simulink model "TFlex_PID"  (R2018a)
settings: Solver=FixedStepDiscrete  StartTime=0.0  StopTime=t_end  FixedStep=ts  RelTol=1e-3
PreLoadFcn:
  | Ts = 0.001;
InitFcn:
  | Ts = 0.001;
values from neighbouring files (symbols this model uses):
  a0 = omega_n^3    (= 31006276.6803)    [Tflex_PID_init.m]
  a1 = 3*omega_n^2    (= 296088.132033)    [Tflex_PID_init.m]
  a2 = 3*omega_n    (= 942.477796077)    [Tflex_PID_init.m]
  b = ones(2*D,Q)*0.001    [Tflex_PID_init.m]
  D = 21    [Tflex_PID_init.m]
  I_limit_max = 500    [Tflex_PID_init.m]
  I_limit_min = -500    [Tflex_PID_init.m]
  Kd = kp*(tau_z-tau_p*(1+(tau_z+tau_p)/tau_i))    [Tflex_PID_init.m]
  Ki = kp/tau_i    [Tflex_PID_init.m]
  Kp = kp*(1+(tau_z-tau_p)/tau_i)    [Tflex_PID_init.m]
  kp = m_eq*crossOver^2/sqrt(1/alpha)    [Tflex_PID_init.m]
  R = eye(2*D,2*D)*sn^2    [Tflex_PID_init.m]
  sf = 185.90    (= 185.9)    [Tflex_PID_init.m]
  t_end = 200    [Tflex_PID_init.m]    (also in multisineInit.m = t(end))
  tau_i = beta*tau_z    [Tflex_PID_init.m]
  tau_p = 1/(crossOver*sqrt(1/alpha))    [Tflex_PID_init.m]
  tau_z = sqrt(1/alpha)/crossOver    [Tflex_PID_init.m]
  ts = 1/1000    (= 0.001)    [Tflex_PID_init.m]    (also in init.m = 0.00025; multisineInit.m)
  w = ones(2*D,Q)*0.001    [Tflex_PID_init.m]
undefined symbols (not defined in the file or in its folder): DiscIntNeverNeededParam, LPden, LPnum, SIGMA
libraries: xpcethercatlib x91, simulink x61, slrtlib x9
(part 2 of 2)

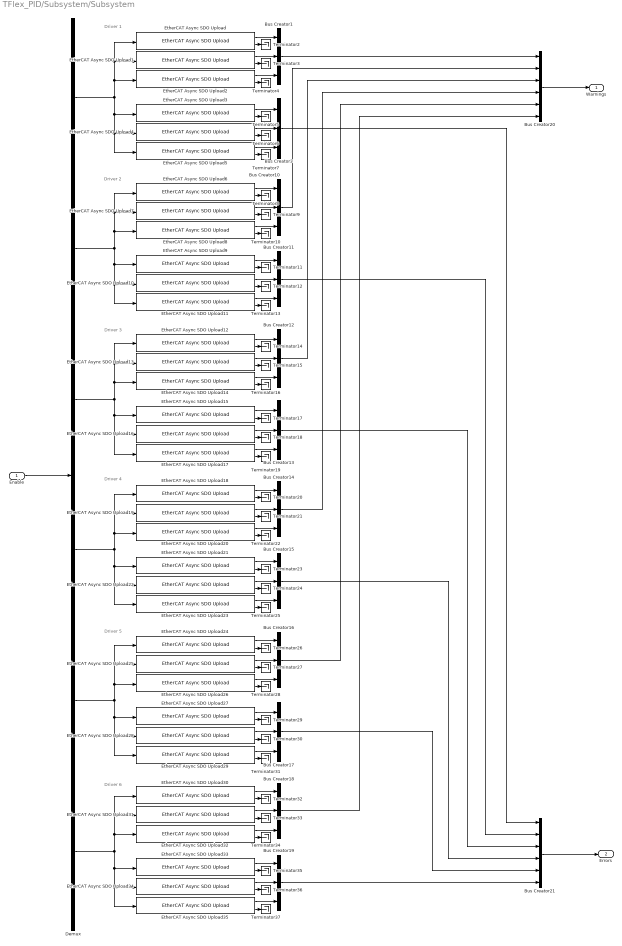
== system TFlex_PID/Subsystem/Subsystem ==
  note: Driver 1
  note: Driver 2
  note: Driver 3
  note: Driver 4
  note: Driver 5
  note: Driver 6
  Enable : Inport
  Bus Creator{1,3,10..19} (12 alike) : BusCreator  Inputs=3
  Bus Creator20 : BusCreator  Inputs=6
  Bus Creator21 : BusCreator  Inputs=6
  Demux : Demux  Outputs=6
  EtherCAT Async SDO Upload : xpcethercatlib/EtherCAT Async SDO Upload  index=8192  subIndex=1  sig_type=uint32  sig_dim=1  device_id=0  slave_name=Drive 2 (AKD)  sample_time=1  slave_addr=1001  selected_slave=Term 1 (EK1100)  timeout=500  slave_found=1
      settings: SourceProductName=Simulink Real-Time  SourceProductBaseCode=XP
  EtherCAT Async SDO Upload1 : xpcethercatlib/EtherCAT Async SDO Upload  index=8192  subIndex=2  sig_type=uint32  sig_dim=1  device_id=0  slave_name=Drive 2 (AKD)  sample_time=1  slave_addr=1001  selected_slave=Term 1 (EK1100)  timeout=500  slave_found=1
      settings: SourceProductName=Simulink Real-Time  SourceProductBaseCode=XP
  EtherCAT Async SDO Upload10 : xpcethercatlib/EtherCAT Async SDO Upload  index=8193  subIndex=2  sig_type=uint32  sig_dim=1  device_id=0  slave_name=Drive 3 (AKD)  sample_time=1  slave_addr=1002  selected_slave=Term 1 (EK1100)  timeout=500  slave_found=1
      settings: SourceProductName=Simulink Real-Time  SourceProductBaseCode=XP
  EtherCAT Async SDO Upload11 : xpcethercatlib/EtherCAT Async SDO Upload  index=8193  subIndex=3  sig_type=uint32  sig_dim=1  device_id=0  slave_name=Drive 3 (AKD)  sample_time=1  slave_addr=1002  selected_slave=Term 1 (EK1100)  timeout=500  slave_found=1
      settings: SourceProductName=Simulink Real-Time  SourceProductBaseCode=XP
  EtherCAT Async SDO Upload12 : xpcethercatlib/EtherCAT Async SDO Upload  index=8192  subIndex=1  sig_type=uint32  sig_dim=1  device_id=0  slave_name=Drive 4 (AKD)  sample_time=1  slave_addr=1003  selected_slave=Term 1 (EK1100)  timeout=500  slave_found=1
      settings: SourceProductName=Simulink Real-Time  SourceProductBaseCode=XP
  EtherCAT Async SDO Upload13 : xpcethercatlib/EtherCAT Async SDO Upload  index=8192  subIndex=2  sig_type=uint32  sig_dim=1  device_id=0  slave_name=Drive 4 (AKD)  sample_time=1  slave_addr=1003  selected_slave=Term 1 (EK1100)  timeout=500  slave_found=1
      settings: SourceProductName=Simulink Real-Time  SourceProductBaseCode=XP
  EtherCAT Async SDO Upload14 : xpcethercatlib/EtherCAT Async SDO Upload  index=8192  subIndex=3  sig_type=uint32  sig_dim=1  device_id=0  slave_name=Drive 4 (AKD)  sample_time=1  slave_addr=1003  selected_slave=Term 1 (EK1100)  timeout=500  slave_found=1
      settings: SourceProductName=Simulink Real-Time  SourceProductBaseCode=XP
  EtherCAT Async SDO Upload15 : xpcethercatlib/EtherCAT Async SDO Upload  index=8193  subIndex=1  sig_type=uint32  sig_dim=1  device_id=0  slave_name=Drive 4 (AKD)  sample_time=1  slave_addr=1003  selected_slave=Term 1 (EK1100)  timeout=500  slave_found=1
      settings: SourceProductName=Simulink Real-Time  SourceProductBaseCode=XP
  EtherCAT Async SDO Upload16 : xpcethercatlib/EtherCAT Async SDO Upload  index=8193  subIndex=2  sig_type=uint32  sig_dim=1  device_id=0  slave_name=Drive 4 (AKD)  sample_time=1  slave_addr=1003  selected_slave=Term 1 (EK1100)  timeout=500  slave_found=1
      settings: SourceProductName=Simulink Real-Time  SourceProductBaseCode=XP
  EtherCAT Async SDO Upload17 : xpcethercatlib/EtherCAT Async SDO Upload  index=8193  subIndex=3  sig_type=uint32  sig_dim=1  device_id=0  slave_name=Drive 4 (AKD)  sample_time=1  slave_addr=1003  selected_slave=Term 1 (EK1100)  timeout=500  slave_found=1
      settings: SourceProductName=Simulink Real-Time  SourceProductBaseCode=XP
  EtherCAT Async SDO Upload18 : xpcethercatlib/EtherCAT Async SDO Upload  index=8192  subIndex=1  sig_type=uint32  sig_dim=1  device_id=0  slave_name=Drive 5 (AKD)  sample_time=1  slave_addr=1004  selected_slave=Term 1 (EK1100)  timeout=500  slave_found=1
      settings: SourceProductName=Simulink Real-Time  SourceProductBaseCode=XP
  EtherCAT Async SDO Upload19 : xpcethercatlib/EtherCAT Async SDO Upload  index=8192  subIndex=2  sig_type=uint32  sig_dim=1  device_id=0  slave_name=Drive 5 (AKD)  sample_time=1  slave_addr=1004  selected_slave=Term 1 (EK1100)  timeout=500  slave_found=1
      settings: SourceProductName=Simulink Real-Time  SourceProductBaseCode=XP
  EtherCAT Async SDO Upload2 : xpcethercatlib/EtherCAT Async SDO Upload  index=8192  subIndex=3  sig_type=uint32  sig_dim=1  device_id=0  slave_name=Drive 1 (AKD)  sample_time=1  slave_addr=1001  selected_slave=Term 1 (EK1100)  timeout=500  slave_found=1
      settings: SourceProductName=Simulink Real-Time  SourceProductBaseCode=XP
  EtherCAT Async SDO Upload20 : xpcethercatlib/EtherCAT Async SDO Upload  index=8192  subIndex=3  sig_type=uint32  sig_dim=1  device_id=0  slave_name=Drive 5 (AKD)  sample_time=1  slave_addr=1004  selected_slave=Term 1 (EK1100)  timeout=500  slave_found=1
      settings: SourceProductName=Simulink Real-Time  SourceProductBaseCode=XP
  EtherCAT Async SDO Upload21 : xpcethercatlib/EtherCAT Async SDO Upload  index=8193  subIndex=1  sig_type=uint32  sig_dim=1  device_id=0  slave_name=Drive 5 (AKD)  sample_time=1  slave_addr=1004  selected_slave=Term 1 (EK1100)  timeout=500  slave_found=1
      settings: SourceProductName=Simulink Real-Time  SourceProductBaseCode=XP
  EtherCAT Async SDO Upload22 : xpcethercatlib/EtherCAT Async SDO Upload  index=8193  subIndex=2  sig_type=uint32  sig_dim=1  device_id=0  slave_name=Drive 5 (AKD)  sample_time=1  slave_addr=1004  selected_slave=Term 1 (EK1100)  timeout=500  slave_found=1
      settings: SourceProductName=Simulink Real-Time  SourceProductBaseCode=XP
  EtherCAT Async SDO Upload23 : xpcethercatlib/EtherCAT Async SDO Upload  index=8193  subIndex=3  sig_type=uint32  sig_dim=1  device_id=0  slave_name=Drive 5 (AKD)  sample_time=1  slave_addr=1004  selected_slave=Term 1 (EK1100)  timeout=500  slave_found=1
      settings: SourceProductName=Simulink Real-Time  SourceProductBaseCode=XP
  EtherCAT Async SDO Upload24 : xpcethercatlib/EtherCAT Async SDO Upload  index=8192  subIndex=1  sig_type=uint32  sig_dim=1  device_id=0  slave_name=Drive 6 (AKD)  sample_time=1  slave_addr=1005  selected_slave=Term 1 (EK1100)  timeout=500  slave_found=1
      settings: SourceProductName=Simulink Real-Time  SourceProductBaseCode=XP
  EtherCAT Async SDO Upload25 : xpcethercatlib/EtherCAT Async SDO Upload  index=8192  subIndex=2  sig_type=uint32  sig_dim=1  device_id=0  slave_name=Drive 6 (AKD)  sample_time=1  slave_addr=1005  selected_slave=Term 1 (EK1100)  timeout=500  slave_found=1
      settings: SourceProductName=Simulink Real-Time  SourceProductBaseCode=XP
  EtherCAT Async SDO Upload26 : xpcethercatlib/EtherCAT Async SDO Upload  index=8192  subIndex=3  sig_type=uint32  sig_dim=1  device_id=0  slave_name=Drive 6 (AKD)  sample_time=1  slave_addr=1005  selected_slave=Term 1 (EK1100)  timeout=500  slave_found=1
      settings: SourceProductName=Simulink Real-Time  SourceProductBaseCode=XP
  EtherCAT Async SDO Upload27 : xpcethercatlib/EtherCAT Async SDO Upload  index=8193  subIndex=1  sig_type=uint32  sig_dim=1  device_id=0  slave_name=Drive 6 (AKD)  sample_time=1  slave_addr=1005  selected_slave=Term 1 (EK1100)  timeout=500  slave_found=1
      settings: SourceProductName=Simulink Real-Time  SourceProductBaseCode=XP
  EtherCAT Async SDO Upload28 : xpcethercatlib/EtherCAT Async SDO Upload  index=8193  subIndex=2  sig_type=uint32  sig_dim=1  device_id=0  slave_name=Drive 6 (AKD)  sample_time=1  slave_addr=1005  selected_slave=Term 1 (EK1100)  timeout=500  slave_found=1
      settings: SourceProductName=Simulink Real-Time  SourceProductBaseCode=XP
  EtherCAT Async SDO Upload29 : xpcethercatlib/EtherCAT Async SDO Upload  index=8193  subIndex=3  sig_type=uint32  sig_dim=1  device_id=0  slave_name=Drive 6 (AKD)  sample_time=1  slave_addr=1005  selected_slave=Term 1 (EK1100)  timeout=500  slave_found=1
      settings: SourceProductName=Simulink Real-Time  SourceProductBaseCode=XP
  EtherCAT Async SDO Upload3 : xpcethercatlib/EtherCAT Async SDO Upload  index=8193  subIndex=1  sig_type=uint32  sig_dim=1  device_id=0  slave_name=""  sample_time=1  slave_addr=0  selected_slave=Term 1 (EK1100)  timeout=500  slave_found=1
      settings: SourceProductName=Simulink Real-Time  SourceProductBaseCode=XP
  EtherCAT Async SDO Upload30 : xpcethercatlib/EtherCAT Async SDO Upload  index=8192  subIndex=1  sig_type=uint32  sig_dim=1  device_id=0  slave_name=Drive 7 (AKD)  sample_time=1  slave_addr=1006  selected_slave=Term 1 (EK1100)  timeout=500  slave_found=1
      settings: SourceProductName=Simulink Real-Time  SourceProductBaseCode=XP
  EtherCAT Async SDO Upload31 : xpcethercatlib/EtherCAT Async SDO Upload  index=8192  subIndex=2  sig_type=uint32  sig_dim=1  device_id=0  slave_name=Drive 7 (AKD)  sample_time=1  slave_addr=1006  selected_slave=Term 1 (EK1100)  timeout=500  slave_found=1
      settings: SourceProductName=Simulink Real-Time  SourceProductBaseCode=XP
  EtherCAT Async SDO Upload32 : xpcethercatlib/EtherCAT Async SDO Upload  index=8192  subIndex=3  sig_type=uint32  sig_dim=1  device_id=0  slave_name=Drive 7 (AKD)  sample_time=1  slave_addr=1006  selected_slave=Term 1 (EK1100)  timeout=500  slave_found=1
      settings: SourceProductName=Simulink Real-Time  SourceProductBaseCode=XP
  EtherCAT Async SDO Upload33 : xpcethercatlib/EtherCAT Async SDO Upload  index=8193  subIndex=1  sig_type=uint32  sig_dim=1  device_id=0  slave_name=Drive 7 (AKD)  sample_time=1  slave_addr=1006  selected_slave=Term 1 (EK1100)  timeout=500  slave_found=1
      settings: SourceProductName=Simulink Real-Time  SourceProductBaseCode=XP
  EtherCAT Async SDO Upload34 : xpcethercatlib/EtherCAT Async SDO Upload  index=8193  subIndex=2  sig_type=uint32  sig_dim=1  device_id=0  slave_name=Drive 7 (AKD)  sample_time=1  slave_addr=1006  selected_slave=Term 1 (EK1100)  timeout=500  slave_found=1
      settings: SourceProductName=Simulink Real-Time  SourceProductBaseCode=XP
  EtherCAT Async SDO Upload35 : xpcethercatlib/EtherCAT Async SDO Upload  index=8193  subIndex=3  sig_type=uint32  sig_dim=1  device_id=0  slave_name=Drive 7 (AKD)  sample_time=1  slave_addr=1006  selected_slave=Term 1 (EK1100)  timeout=500  slave_found=1
      settings: SourceProductName=Simulink Real-Time  SourceProductBaseCode=XP
  EtherCAT Async SDO Upload4 : xpcethercatlib/EtherCAT Async SDO Upload  index=8193  subIndex=2  sig_type=uint32  sig_dim=1  device_id=0  slave_name=Drive 2 (AKD)  sample_time=1  slave_addr=1001  selected_slave=Term 1 (EK1100)  timeout=500  slave_found=1
      settings: SourceProductName=Simulink Real-Time  SourceProductBaseCode=XP
  EtherCAT Async SDO Upload5 : xpcethercatlib/EtherCAT Async SDO Upload  index=8193  subIndex=3  sig_type=uint32  sig_dim=1  device_id=0  slave_name=Drive 1 (AKD)  sample_time=1  slave_addr=1001  selected_slave=Term 1 (EK1100)  timeout=500  slave_found=1
      settings: SourceProductName=Simulink Real-Time  SourceProductBaseCode=XP
  EtherCAT Async SDO Upload6 : xpcethercatlib/EtherCAT Async SDO Upload  index=8192  subIndex=1  sig_type=uint32  sig_dim=1  device_id=0  slave_name=Drive 3 (AKD)  sample_time=1  slave_addr=1002  selected_slave=Term 1 (EK1100)  timeout=500  slave_found=1
      settings: SourceProductName=Simulink Real-Time  SourceProductBaseCode=XP
  EtherCAT Async SDO Upload7 : xpcethercatlib/EtherCAT Async SDO Upload  index=8192  subIndex=2  sig_type=uint32  sig_dim=1  device_id=0  slave_name=Drive 3 (AKD)  sample_time=1  slave_addr=1002  selected_slave=Term 1 (EK1100)  timeout=500  slave_found=1
      settings: SourceProductName=Simulink Real-Time  SourceProductBaseCode=XP
  EtherCAT Async SDO Upload8 : xpcethercatlib/EtherCAT Async SDO Upload  index=8192  subIndex=3  sig_type=uint32  sig_dim=1  device_id=0  slave_name=Drive 3 (AKD)  sample_time=1  slave_addr=1002  selected_slave=Term 1 (EK1100)  timeout=500  slave_found=1
      settings: SourceProductName=Simulink Real-Time  SourceProductBaseCode=XP
  EtherCAT Async SDO Upload9 : xpcethercatlib/EtherCAT Async SDO Upload  index=8193  subIndex=1  sig_type=uint32  sig_dim=1  device_id=0  slave_name=Drive 3 (AKD)  sample_time=1  slave_addr=1002  selected_slave=Term 1 (EK1100)  timeout=500  slave_found=1
      settings: SourceProductName=Simulink Real-Time  SourceProductBaseCode=XP
  Terminator{2..37} (36 alike) : Terminator
  Warnings : Outport
  Errors : Outport  Port=2
  wires:
  EtherCAT Async SDO Upload13/2 -> Terminator15/1
  EtherCAT Async SDO Upload23/2 -> Terminator25/1
  EtherCAT Async SDO Upload25/2 -> Terminator27/1
  EtherCAT Async SDO Upload9/2 -> Terminator11/1
  EtherCAT Async SDO Upload5/2 -> Terminator7/1
  EtherCAT Async SDO Upload30/2 -> Terminator32/1
  EtherCAT Async SDO Upload27/2 -> Terminator29/1
  EtherCAT Async SDO Upload12/2 -> Terminator14/1
  EtherCAT Async SDO Upload24/2 -> Terminator26/1
  EtherCAT Async SDO Upload26/2 -> Terminator28/1
  Bus Creator12/1 -> Bus Creator20/3
  Demux/3 -> EtherCAT Async SDO Upload12/1, EtherCAT Async SDO Upload13/1, EtherCAT Async SDO Upload14/1, EtherCAT Async SDO Upload17/1, EtherCAT Async SDO Upload16/1, EtherCAT Async SDO Upload15/1
  EtherCAT Async SDO Upload30/1 -> Bus Creator18/1
  Demux/2 -> EtherCAT Async SDO Upload11/1, EtherCAT Async SDO Upload10/1, EtherCAT Async SDO Upload9/1, EtherCAT Async SDO Upload6/1, EtherCAT Async SDO Upload7/1, EtherCAT Async SDO Upload8/1
  EtherCAT Async SDO Upload9/1 -> Bus Creator11/1
  EtherCAT Async SDO Upload18/2 -> Terminator20/1
  EtherCAT Async SDO Upload8/2 -> Terminator10/1
  EtherCAT Async SDO Upload11/2 -> Terminator13/1
  Demux/6 -> EtherCAT Async SDO Upload30/1, EtherCAT Async SDO Upload31/1, EtherCAT Async SDO Upload32/1, EtherCAT Async SDO Upload35/1, EtherCAT Async SDO Upload34/1, EtherCAT Async SDO Upload33/1
  Demux/4 -> EtherCAT Async SDO Upload18/1, EtherCAT Async SDO Upload19/1, EtherCAT Async SDO Upload20/1, EtherCAT Async SDO Upload23/1, EtherCAT Async SDO Upload22/1, EtherCAT Async SDO Upload21/1
  EtherCAT Async SDO Upload19/2 -> Terminator21/1
  Bus Creator19/1 -> Bus Creator21/6
  Demux/1 -> EtherCAT Async SDO Upload5/1, EtherCAT Async SDO Upload4/1, EtherCAT Async SDO Upload3/1, EtherCAT Async SDO Upload/1, EtherCAT Async SDO Upload1/1, EtherCAT Async SDO Upload2/1
  EtherCAT Async SDO Upload15/2 -> Terminator17/1
  Bus Creator14/1 -> Bus Creator20/4
  EtherCAT Async SDO Upload34/2 -> Terminator36/1
  Demux/5 -> EtherCAT Async SDO Upload24/1, EtherCAT Async SDO Upload25/1, EtherCAT Async SDO Upload26/1, EtherCAT Async SDO Upload29/1, EtherCAT Async SDO Upload28/1, EtherCAT Async SDO Upload27/1
  EtherCAT Async SDO Upload6/2 -> Terminator8/1
  EtherCAT Async SDO Upload/1 -> Bus Creator1/1
  EtherCAT Async SDO Upload7/2 -> Terminator9/1
  EtherCAT Async SDO Upload16/2 -> Terminator18/1
  Bus Creator13/1 -> Bus Creator21/3
  EtherCAT Async SDO Upload10/2 -> Terminator12/1
  EtherCAT Async SDO Upload35/2 -> Terminator37/1
  EtherCAT Async SDO Upload21/1 -> Bus Creator15/1
  Bus Creator16/1 -> Bus Creator20/5
  EtherCAT Async SDO Upload31/2 -> Terminator33/1
  EtherCAT Async SDO Upload32/1 -> Bus Creator18/3
  EtherCAT Async SDO Upload15/1 -> Bus Creator13/1
  EtherCAT Async SDO Upload/2 -> Terminator2/1
  EtherCAT Async SDO Upload13/1 -> Bus Creator12/2
  EtherCAT Async SDO Upload33/2 -> Terminator35/1
  EtherCAT Async SDO Upload4/2 -> Terminator6/1
  EtherCAT Async SDO Upload28/2 -> Terminator30/1
  EtherCAT Async SDO Upload1/2 -> Terminator3/1
  Bus Creator10/1 -> Bus Creator20/2
  EtherCAT Async SDO Upload8/1 -> Bus Creator10/3
  EtherCAT Async SDO Upload19/1 -> Bus Creator14/2
  EtherCAT Async SDO Upload20/2 -> Terminator22/1
  EtherCAT Async SDO Upload12/1 -> Bus Creator12/1
  EtherCAT Async SDO Upload29/2 -> Terminator31/1
  EtherCAT Async SDO Upload2/1 -> Bus Creator1/3
  EtherCAT Async SDO Upload26/1 -> Bus Creator16/3
  EtherCAT Async SDO Upload22/2 -> Terminator24/1
  EtherCAT Async SDO Upload28/1 -> Bus Creator17/2
  Bus Creator1/1 -> Bus Creator20/1
  EtherCAT Async SDO Upload3/2 -> Terminator5/1
  Bus Creator17/1 -> Bus Creator21/5
  EtherCAT Async SDO Upload2/2 -> Terminator4/1
  EtherCAT Async SDO Upload33/1 -> Bus Creator19/1
  EtherCAT Async SDO Upload17/1 -> Bus Creator13/3
  EtherCAT Async SDO Upload31/1 -> Bus Creator18/2
  EtherCAT Async SDO Upload27/1 -> Bus Creator17/1
  EtherCAT Async SDO Upload1/1 -> Bus Creator1/2
  EtherCAT Async SDO Upload3/1 -> Bus Creator3/1
  EtherCAT Async SDO Upload11/1 -> Bus Creator11/3
  EtherCAT Async SDO Upload7/1 -> Bus Creator10/2
  EtherCAT Async SDO Upload6/1 -> Bus Creator10/1
  EtherCAT Async SDO Upload34/1 -> Bus Creator19/2
  Bus Creator18/1 -> Bus Creator20/6
  EtherCAT Async SDO Upload22/1 -> Bus Creator15/2
  EtherCAT Async SDO Upload23/1 -> Bus Creator15/3
  EtherCAT Async SDO Upload18/1 -> Bus Creator14/1
  EtherCAT Async SDO Upload10/1 -> Bus Creator11/2
  EtherCAT Async SDO Upload14/1 -> Bus Creator12/3
  EtherCAT Async SDO Upload35/1 -> Bus Creator19/3
  EtherCAT Async SDO Upload24/1 -> Bus Creator16/1
  EtherCAT Async SDO Upload20/1 -> Bus Creator14/3
  Bus Creator3/1 -> Bus Creator21/1
  EtherCAT Async SDO Upload4/1 -> Bus Creator3/2
  EtherCAT Async SDO Upload25/1 -> Bus Creator16/2
  EtherCAT Async SDO Upload16/1 -> Bus Creator13/2
  Bus Creator15/1 -> Bus Creator21/4
  Bus Creator11/1 -> Bus Creator21/2
  EtherCAT Async SDO Upload5/1 -> Bus Creator3/3
  EtherCAT Async SDO Upload32/2 -> Terminator34/1
  EtherCAT Async SDO Upload29/1 -> Bus Creator17/3
  EtherCAT Async SDO Upload14/2 -> Terminator16/1
  EtherCAT Async SDO Upload17/2 -> Terminator19/1
  EtherCAT Async SDO Upload21/2 -> Terminator23/1
  Bus Creator21/1 -> Errors/1
  Bus Creator20/1 -> Warnings/1
  Enable/1 -> Demux/1

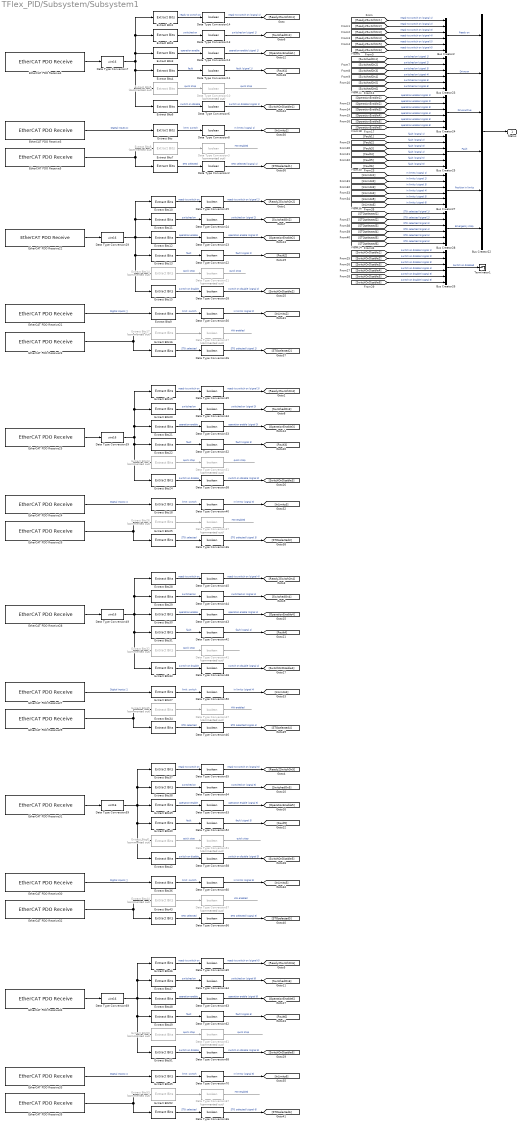
== system TFlex_PID/Subsystem/Subsystem1 ==
  Bus Creator2 : BusCreator  Inputs=ready to switch on (signal 1),ready to switch on (signal 2),ready to switch on (signal 3),ready to switch on (signal 4),ready to switch on (signal 5),ready to switch on (signal 6)
  Bus Creator22 : BusCreator  Inputs=Ready on,Drive on,Drive active,Fault,Position in limits,Emergency stop
  Bus Creator23 : BusCreator  Inputs=switched on (signal 1),switched on (signal 2),switched on (signal 3),switched on (signal 4),switched on (signal 5),switched on (signal 6)
  Bus Creator24 : BusCreator  Inputs=operation enable (signal 1),operation enable (signal 2),operation enable (signal 3),operation enable (signal 4),operation enable (signal 5),operation enable (signal 6)
  Bus Creator25 : BusCreator  Inputs=fault (signal 1),fault (signal 2),fault (signal 3),fault (signal 4),fault (signal 5),fault (signal 6)
  Bus Creator26 : BusCreator  Inputs=switch on disable (signal 1),switch on disable (signal 2),switch on disable (signal 3),switch on disable (signal 4),switch on disable (signal 5),switch on disable (signal 6)
  Bus Creator27 : BusCreator  Inputs=in limits (signal 1),in limits (signal 2),in limits (signal 3),in limits (signal 4),in limits (signal 5),in limits (signal 6)
  Bus Creator28 : BusCreator  Inputs=STO selected (signal 1),STO selected (signal 2),STO selected (signal 3),STO selected (signal 4),STO selected (signal 5),STO selected (signal 6)
  Data Type Conversion{3,10,21,27,31,37,41,47,51,57,61,67} (12 alike) : DataTypeConversion  Commented=on  OutDataTypeStr=boolean
  Data Type Conversion{2,6,8,11..14,22..26,28,30,32..36,38,40,42..46,48,50,52..56,58,60,62..66,68,70} (42 alike) : DataTypeConversion  OutDataTypeStr=boolean
  Data Type Conversion{7,29,39,49,59,69} (6 alike) : DataTypeConversion  OutDataTypeStr=uint16  RndMeth=Round
  EtherCAT PDO Receive21 : xpcethercatlib/EtherCAT PDO Receive  Priority=2  sig_name=Drive 3 (AKD).Inputs.Digital inputs  sig_offset=12528  sig_type=uint32  type_size=32  sig_dim=1  device_id=0  sample_time=0.001000
      settings: SourceProductName=Simulink Real-Time  SourceProductBaseCode=XP
  EtherCAT PDO Receive22 : xpcethercatlib/EtherCAT PDO Receive  Priority=2  sig_name=Drive 3 (AKD).Inputs.Statusword  sig_offset=12496  sig_type=uint16  type_size=16  sig_dim=1  device_id=0  sample_time=0.001000
      settings: SourceProductName=Simulink Real-Time  SourceProductBaseCode=XP
  EtherCAT PDO Receive23 : xpcethercatlib/EtherCAT PDO Receive  Priority=2  sig_name=Drive 3 (AKD).Inputs_2.Manufacturer status register  sig_offset=12624  sig_type=uint32  type_size=32  sig_dim=1  device_id=0  sample_time=0.001000
      settings: SourceProductName=Simulink Real-Time  SourceProductBaseCode=XP
  EtherCAT PDO Receive24 : xpcethercatlib/EtherCAT PDO Receive  Priority=2  sig_name=Drive 4 (AKD).Inputs.Digital inputs  sig_offset=24816  sig_type=uint32  type_size=32  sig_dim=1  device_id=0  sample_time=0.001000
      settings: SourceProductName=Simulink Real-Time  SourceProductBaseCode=XP
  EtherCAT PDO Receive25 : xpcethercatlib/EtherCAT PDO Receive  Priority=2  sig_name=Drive 4 (AKD).Inputs.Statusword  sig_offset=24784  sig_type=uint16  type_size=16  sig_dim=1  device_id=0  sample_time=0.001000
      settings: SourceProductName=Simulink Real-Time  SourceProductBaseCode=XP
  EtherCAT PDO Receive26 : xpcethercatlib/EtherCAT PDO Receive  Priority=2  sig_name=Drive 4 (AKD).Inputs_2.Manufacturer status register  sig_offset=24912  sig_type=uint32  type_size=32  sig_dim=1  device_id=0  sample_time=0.001000
      settings: SourceProductName=Simulink Real-Time  SourceProductBaseCode=XP
  EtherCAT PDO Receive27 : xpcethercatlib/EtherCAT PDO Receive  Priority=2  sig_name=Drive 5 (AKD).Inputs.Digital inputs  sig_offset=37104  sig_type=uint32  type_size=32  sig_dim=1  device_id=0  sample_time=0.001000
      settings: SourceProductName=Simulink Real-Time  SourceProductBaseCode=XP
  EtherCAT PDO Receive28 : xpcethercatlib/EtherCAT PDO Receive  Priority=2  sig_name=Drive 5 (AKD).Inputs.Statusword  sig_offset=37072  sig_type=uint16  type_size=16  sig_dim=1  device_id=0  sample_time=0.001000
      settings: SourceProductName=Simulink Real-Time  SourceProductBaseCode=XP
  EtherCAT PDO Receive29 : xpcethercatlib/EtherCAT PDO Receive  Priority=2  sig_name=Drive 5 (AKD).Inputs_2.Manufacturer status register  sig_offset=37200  sig_type=uint32  type_size=32  sig_dim=1  device_id=0  sample_time=0.001000
      settings: SourceProductName=Simulink Real-Time  SourceProductBaseCode=XP
  EtherCAT PDO Receive3 : xpcethercatlib/EtherCAT PDO Receive  Priority=2  sig_name=Drive 2 (AKD).Inputs.Digital inputs  sig_offset=496  sig_type=uint32  type_size=32  sig_dim=1  device_id=0  sample_time=0.001000
      settings: SourceProductName=Simulink Real-Time  SourceProductBaseCode=XP
  EtherCAT PDO Receive30 : xpcethercatlib/EtherCAT PDO Receive  Priority=2  sig_name=Drive 6 (AKD).Inputs.Digital inputs  sig_offset=37264  sig_type=uint32  type_size=32  sig_dim=1  device_id=0  sample_time=0.001000
      settings: SourceProductName=Simulink Real-Time  SourceProductBaseCode=XP
  EtherCAT PDO Receive31 : xpcethercatlib/EtherCAT PDO Receive  Priority=2  sig_name=Drive 6 (AKD).Inputs.Statusword  sig_offset=37232  sig_type=uint16  type_size=16  sig_dim=1  device_id=0  sample_time=0.001000
      settings: SourceProductName=Simulink Real-Time  SourceProductBaseCode=XP
  EtherCAT PDO Receive32 : xpcethercatlib/EtherCAT PDO Receive  Priority=2  sig_name=Drive 6 (AKD).Inputs_2.Manufacturer status register  sig_offset=37360  sig_type=uint32  type_size=32  sig_dim=1  device_id=0  sample_time=0.001000
      settings: SourceProductName=Simulink Real-Time  SourceProductBaseCode=XP
  EtherCAT PDO Receive33 : xpcethercatlib/EtherCAT PDO Receive  Priority=2  sig_name=Drive 7 (AKD).Inputs.Digital inputs  sig_offset=37424  sig_type=uint32  type_size=32  sig_dim=1  device_id=0  sample_time=0.001000
      settings: SourceProductName=Simulink Real-Time  SourceProductBaseCode=XP
  EtherCAT PDO Receive34 : xpcethercatlib/EtherCAT PDO Receive  Priority=2  sig_name=Drive 7 (AKD).Inputs.Statusword  sig_offset=37392  sig_type=uint16  type_size=16  sig_dim=1  device_id=0  sample_time=0.001000
      settings: SourceProductName=Simulink Real-Time  SourceProductBaseCode=XP
  EtherCAT PDO Receive35 : xpcethercatlib/EtherCAT PDO Receive  Priority=2  sig_name=Drive 7 (AKD).Inputs_2.Manufacturer status register  sig_offset=37520  sig_type=uint32  type_size=32  sig_dim=1  device_id=0  sample_time=0.001000
      settings: SourceProductName=Simulink Real-Time  SourceProductBaseCode=XP
  EtherCAT PDO Receive4 : xpcethercatlib/EtherCAT PDO Receive  Priority=2  sig_name=Drive 2 (AKD).Inputs.Statusword  sig_offset=464  sig_type=uint16  type_size=16  sig_dim=1  device_id=0  sample_time=0.001000
      settings: SourceProductName=Simulink Real-Time  SourceProductBaseCode=XP
  EtherCAT PDO Receive5 : xpcethercatlib/EtherCAT PDO Receive  Priority=2  sig_name=Drive 2 (AKD).Inputs_2.Manufacturer status register  sig_offset=592  sig_type=uint32  type_size=32  sig_dim=1  device_id=0  sample_time=0.001000
      settings: SourceProductName=Simulink Real-Time  SourceProductBaseCode=XP
  Extract Bits{,9,18,27,36,45} (6 alike) : simulink/Logic and Bit Operations/Extract Bits  bitsToExtract=Range of bits  numBits=8  bitIdxRange=[16]  outScalingMode=Treat bit field as an integer
      settings: SourceProductName=Simulink
  Extract Bits{1,10,19,28,37,46} (6 alike) : simulink/Logic and Bit Operations/Extract Bits  bitsToExtract=Range of bits  numBits=8  bitIdxRange=[0]  outScalingMode=Treat bit field as an integer
      settings: SourceProductName=Simulink
  Extract Bits{2,11,20,29,38,47} (6 alike) : simulink/Logic and Bit Operations/Extract Bits  bitsToExtract=Range of bits  numBits=8  bitIdxRange=[1]  outScalingMode=Treat bit field as an integer
      settings: SourceProductName=Simulink
  Extract Bits{3,12,21,30,39,48} (6 alike) : simulink/Logic and Bit Operations/Extract Bits  bitsToExtract=Range of bits  numBits=8  bitIdxRange=[2]  outScalingMode=Treat bit field as an integer
      settings: SourceProductName=Simulink
  Extract Bits{4,13,22,31,40,49} (6 alike) : simulink/Logic and Bit Operations/Extract Bits  bitsToExtract=Range of bits  numBits=8  bitIdxRange=[3]  outScalingMode=Treat bit field as an integer
      settings: SourceProductName=Simulink
  Extract Bits{5,14,23,32,41,50} (6 alike) : simulink/Logic and Bit Operations/Extract Bits  Commented=on  bitsToExtract=Range of bits  numBits=8  bitIdxRange=[5]  outScalingMode=Treat bit field as an integer
      settings: SourceProductName=Simulink
  Extract Bits{6,15,24,33,42,51} (6 alike) : simulink/Logic and Bit Operations/Extract Bits  bitsToExtract=Range of bits  numBits=8  bitIdxRange=[6]  outScalingMode=Treat bit field as an integer
      settings: SourceProductName=Simulink
  Extract Bits{7,16,25,34,43,52} (6 alike) : simulink/Logic and Bit Operations/Extract Bits  bitsToExtract=Range of bits  numBits=8  bitIdxRange=[13]  outScalingMode=Treat bit field as an integer
      settings: SourceProductName=Simulink
  Extract Bits{8,17,26,35,44,53} (6 alike) : simulink/Logic and Bit Operations/Extract Bits  Commented=on  bitsToExtract=Range of bits  numBits=8  bitIdxRange=[29]  outScalingMode=Treat bit field as an integer
      settings: SourceProductName=Simulink
  Terminator1 : Terminator
  Status : Outport
  wires:
  EtherCAT PDO Receive27/1 -> Extract Bits27/1  "Digital inputs []"
  [OperationEnable1] -> Bus Creator24/1  "operation enable (signal 1)"
  Data Type Conversion49/1 -> Extract Bits30/1, Extract Bits31/1, Extract Bits33/1, Extract Bits32/1, Extract Bits28/1, Extract Bits29/1
  [SwitchOnDisable3] -> Bus Creator26/3  "switch on disable (signal 3)"
  Data Type Conversion60/1 -> [InLimits5]  "in limits (signal 5)"
  EtherCAT PDO Receive26/1 -> Extract Bits26/1, Extract Bits25/1
  [OperationEnable2] -> Bus Creator24/2  "operation enable (signal 2)"
  [Fault2] -> Bus Creator25/2  "fault (signal 2)"
  Data Type Conversion31/1 -> ?  "quick stop"
  Data Type Conversion39/1 -> Extract Bits22/1, Extract Bits23/1, Extract Bits24/1, Extract Bits21/1, Extract Bits19/1, Extract Bits20/1
  Data Type Conversion69/1 -> Extract Bits51/1, Extract Bits50/1, Extract Bits49/1, Extract Bits46/1, Extract Bits47/1, Extract Bits48/1
  EtherCAT PDO Receive31/1 -> Data Type Conversion59/1
  Data Type Conversion68/1 -> [SwitchOnDisable6]  "switch on disable (signal 6)"
  [Ready2SwitchOn2] -> Bus Creator2/2  "ready to switch on (signal 2)"
  Extract Bits8/1 -> Data Type Conversion3/1
  Data Type Conversion7/1 -> Extract Bits1/1, Extract Bits2/1, Extract Bits3/1, Extract Bits6/1, Extract Bits5/1, Extract Bits4/1
  [SwitchOnDisable1] -> Bus Creator26/1  "switch on disable (signal 1)"
  Data Type Conversion50/1 -> [InLimits4]  "in limits (signal 4)"
  Data Type Conversion29/1 -> Extract Bits15/1, Extract Bits14/1, Extract Bits13/1, Extract Bits10/1, Extract Bits11/1, Extract Bits12/1
  Data Type Conversion51/1 -> ?  "quick stop"
  [STOselected4] -> Bus Creator28/4  "STO selected (signal 4)"
  Data Type Conversion13/1 -> [SwitchedOn1]  "switched on (signal 1)"
  Data Type Conversion43/1 -> [OperationEnable4]  "operation enable (signal 4)"
  Extract Bits44/1 -> Data Type Conversion57/1
  Bus Creator2/1 -> Bus Creator22/1  "Ready on"
  Extract Bits5/1 -> Data Type Conversion10/1  "quick stop"
  Data Type Conversion59/1 -> Extract Bits42/1, Extract Bits41/1, Extract Bits40/1, Extract Bits37/1, Extract Bits38/1, Extract Bits39/1
  Extract Bits24/1 -> Data Type Conversion38/1  "switch on disable"
  Data Type Conversion26/1 -> [STOselected2]  "STO selected (signal 2)"
  EtherCAT PDO Receive29/1 -> Extract Bits34/1, Extract Bits35/1
  Data Type Conversion63/1 -> [OperationEnable6]  "operation enable (signal 6)"
  Extract Bits36/1 -> Data Type Conversion60/1  "limit  switch"
  [Ready2SwitchOn5] -> Bus Creator2/5  "ready to switch on (signal 5)"
  Extract Bits35/1 -> Data Type Conversion47/1
  Data Type Conversion11/1 -> [Fault1]  "fault (signal 1)"
  Data Type Conversion58/1 -> [SwitchOnDisable5]  "switch on disable (signal 5)"
  Extract Bits48/1 -> Data Type Conversion63/1  "operation enable"
  Data Type Conversion35/1 -> [Ready2SwitchOn3]  "ready to switch on (signal 3)"
  EtherCAT PDO Receive23/1 -> Extract Bits17/1, Extract Bits16/1
  Data Type Conversion55/1 -> [Ready2SwitchOn5]  "ready to switch on (signal 5)"
  [Fault6] -> Bus Creator25/6  "fault (signal 6)"
  [SwitchedOn3] -> Bus Creator23/3  "switched on (signal 3)"
  Data Type Conversion54/1 -> [SwitchedOn5]  "switched on (signal 5)"
  [InLimits3] -> Bus Creator27/3  "in limits (signal 3)"
  Data Type Conversion2/1 -> [STOselected1]  "STO selected (signal 1)"
  [STOselected6] -> Bus Creator28/6  "STO selected (signal 6)"
  Extract Bits46/1 -> Data Type Conversion65/1  "ready to switch on"
  [SwitchOnDisable2] -> Bus Creator26/2  "switch on disable (signal 2)"
  Data Type Conversion64/1 -> [SwitchedOn6]  "switched on (signal 6)"
  [InLimits4] -> Bus Creator27/4  "in limits (signal 4)"
  Data Type Conversion70/1 -> [InLimits6]  "in limits (signal 6)"
  [SwitchedOn5] -> Bus Creator23/5  "switched on (signal 5)"
  [STOselected5] -> Bus Creator28/5  "STO selected (signal 5)"
  [InLimits6] -> Bus Creator27/6  "in limits (signal 6)"
  EtherCAT PDO Receive32/1 -> Extract Bits43/1, Extract Bits44/1
  Data Type Conversion65/1 -> [Ready2SwitchOn6]  "ready to switch on (signal 6)"
  [OperationEnable3] -> Bus Creator24/3  "operation enable (signal 3)"
  Data Type Conversion48/1 -> [SwitchOnDisable4]  "switch on disable (signal 4)"
  Data Type Conversion32/1 -> [Fault3]  "fault (signal 3)"
  Data Type Conversion46/1 -> [STOselected4]  "STO selected (signal 4)"
  Data Type Conversion38/1 -> [SwitchOnDisable3]  "switch on disable (signal 3)"
  Data Type Conversion23/1 -> [OperationEnable2]  "operation enable (signal 2)"
  Extract Bits39/1 -> Data Type Conversion53/1  "operation enable"
  [SwitchedOn4] -> Bus Creator23/4  "switched on (signal 4)"
  Extract Bits38/1 -> Data Type Conversion54/1  "switched on"
  [STOselected2] -> Bus Creator28/2  "STO selected (signal 2)"
  Data Type Conversion34/1 -> [SwitchedOn3]  "switched on (signal 3)"
  Extract Bits3/1 -> Data Type Conversion12/1  "operation enable"
  Data Type Conversion45/1 -> [Ready2SwitchOn4]  "ready to switch on (signal 4)"
  Extract Bits43/1 -> Data Type Conversion56/1  "STO selected"
  Data Type Conversion8/1 -> [InLimits1]  "in limits (signal 1)"
  [Ready2SwitchOn4] -> Bus Creator2/4  "ready to switch on (signal 4)"
  [STOselected3] -> Bus Creator28/3  "STO selected (signal 3)"
  [STOselected1] -> Bus Creator28/1  "STO selected (signal 1)"
  [InLimits5] -> Bus Creator27/5  "in limits (signal 5)"
  Bus Creator27/1 -> Bus Creator22/5  "Position in limits"
  Data Type Conversion33/1 -> [OperationEnable3]  "operation enable (signal 3)"
  Extract Bits14/1 -> Data Type Conversion21/1  "quick stop"
  Extract Bits45/1 -> Data Type Conversion70/1  "limit  switch"
  [Fault1] -> Bus Creator25/1  "fault (signal 1)"
  EtherCAT PDO Receive4/1 -> Data Type Conversion7/1
  Data Type Conversion40/1 -> [InLimits3]  "in limits (signal 3)"
  Extract Bits47/1 -> Data Type Conversion64/1  "switched on"
  [SwitchedOn2] -> Bus Creator23/2  "switched on (signal 2)"
  Data Type Conversion12/1 -> [OperationEnable1]  "operation enable (signal 1)"
  [Ready2SwitchOn6] -> Bus Creator2/6  "ready to switch on (signal 6)"
  Data Type Conversion42/1 -> [Fault4]  "fault (signal 4)"
  [Ready2SwitchOn3] -> Bus Creator2/3  "ready to switch on (signal 3)"
  [SwitchedOn6] -> Bus Creator23/6  "switched on (signal 6)"
  [SwitchOnDisable6] -> Bus Creator26/6  "switch on disable (signal 6)"
  [SwitchOnDisable5] -> Bus Creator26/5  "switch on disable (signal 5)"
  Data Type Conversion22/1 -> [Fault2]  "fault (signal 2)"
  Data Type Conversion24/1 -> [SwitchedOn2]  "switched on (signal 2)"
  Data Type Conversion53/1 -> [OperationEnable5]  "operation enable (signal 5)"
  Extract Bits22/1 -> Data Type Conversion32/1  "fault"
  Extract Bits23/1 -> Data Type Conversion31/1  "quick stop"
  [Ready2SwitchOn1] -> Bus Creator2/1  "ready to switch on (signal 1)"
  EtherCAT PDO Receive28/1 -> Data Type Conversion49/1
  Data Type Conversion25/1 -> [Ready2SwitchOn2]  "ready to switch on (signal 2)"
  Extract Bits52/1 -> Data Type Conversion66/1  "STO selected"
  [OperationEnable6] -> Bus Creator24/6  "operation enable (signal 6)"
  Data Type Conversion14/1 -> [Ready2SwitchOn1]  "ready to switch on (signal 1)"
  Extract Bits33/1 -> Data Type Conversion48/1  "switch on disable"
  Data Type Conversion28/1 -> [SwitchOnDisable2]  "switch on disable (signal 2)"
  Data Type Conversion62/1 -> [Fault6]  "fault (signal 6)"
  EtherCAT PDO Receive5/1 -> Extract Bits7/1, Extract Bits8/1
  Data Type Conversion30/1 -> [InLimits2]  "in limits (signal 2)"
  [Fault3] -> Bus Creator25/3  "fault (signal 3)"
  EtherCAT PDO Receive33/1 -> Extract Bits45/1  "Digital inputs []"
  Data Type Conversion36/1 -> [STOselected3]  "STO selected (signal 3)"
  Data Type Conversion66/1 -> [STOselected6]  "STO selected (signal 6)"
  EtherCAT PDO Receive35/1 -> Extract Bits52/1, Extract Bits53/1
  Data Type Conversion44/1 -> [SwitchedOn4]  "switched on (signal 4)"
  Data Type Conversion6/1 -> [SwitchOnDisable1]  "switch on disable (signal 1)"
  [Fault5] -> Bus Creator25/5  "fault (signal 5)"
  [Fault4] -> Bus Creator25/4  "fault (signal 4)"
  Extract Bits25/1 -> Data Type Conversion36/1  "STO selected"
  Bus Creator24/1 -> Bus Creator22/3  "Drive active"
  [SwitchedOn1] -> Bus Creator23/1  "switched on (signal 1)"
  Data Type Conversion52/1 -> [Fault5]  "fault (signal 5)"
  [OperationEnable5] -> Bus Creator24/5  "operation enable (signal 5)"
  Extract Bits15/1 -> Data Type Conversion28/1  "switch on disable"
  Data Type Conversion56/1 -> [STOselected5]  "STO selected (signal 5)"
  [SwitchOnDisable4] -> Bus Creator26/4  "switch on disable (signal 4)"
  Extract Bits16/1 -> Data Type Conversion26/1  "STO selected"
  [InLimits1] -> Bus Creator27/1  "in limits (signal 1)"
  [InLimits2] -> Bus Creator27/2  "in limits (signal 2)"
  [OperationEnable4] -> Bus Creator24/4  "operation enable (signal 4)"
  EtherCAT PDO Receive34/1 -> Data Type Conversion69/1
  Extract Bits26/1 -> Data Type Conversion37/1
  Bus Creator26/1 -> Terminator1/1  "Switch on disabled"
  Extract Bits29/1 -> Data Type Conversion44/1  "switched on"
  EtherCAT PDO Receive30/1 -> Extract Bits36/1  "Digital inputs []"
  Extract Bits11/1 -> Data Type Conversion24/1  "switched on"
  Data Type Conversion27/1 -> ?  "HW enabled"
  EtherCAT PDO Receive24/1 -> Extract Bits18/1  "Digital inputs []"
  Extract Bits42/1 -> Data Type Conversion58/1  "switch on disable"
  Extract Bits51/1 -> Data Type Conversion68/1  "switch on disable"
  Bus Creator28/1 -> Bus Creator22/6  "Emergency stop"
  Extract Bits41/1 -> Data Type Conversion51/1  "quick stop"
  Extract Bits2/1 -> Data Type Conversion13/1  "switched on"
  Extract Bits31/1 -> Data Type Conversion42/1  "fault"
  Extract Bits30/1 -> Data Type Conversion43/1  "operation enable"
  Extract Bits10/1 -> Data Type Conversion25/1  "ready to switch on"
  Extract Bits19/1 -> Data Type Conversion35/1  "ready to switch on"
  Extract Bits20/1 -> Data Type Conversion34/1  "switched on"
  Extract Bits37/1 -> Data Type Conversion55/1  "ready to switch on"
  Extract Bits12/1 -> Data Type Conversion23/1  "operation enable"
  Extract Bits18/1 -> Data Type Conversion40/1  "limit  switch"
  EtherCAT PDO Receive21/1 -> Extract Bits9/1  "Digital inputs []"
  EtherCAT PDO Receive25/1 -> Data Type Conversion39/1
  Extract Bits32/1 -> Data Type Conversion41/1  "quick stop"
  Extract Bits6/1 -> Data Type Conversion6/1  "switch on disable"
  Extract Bits53/1 -> Data Type Conversion67/1
  Extract Bits27/1 -> Data Type Conversion50/1  "limit  switch"
  Extract Bits1/1 -> Data Type Conversion14/1  "ready to switch on"
  Extract Bits21/1 -> Data Type Conversion33/1  "operation enable"
  Bus Creator23/1 -> Bus Creator22/2  "Drive on"
  Extract Bits34/1 -> Data Type Conversion46/1  "STO selected"
  Extract Bits4/1 -> Data Type Conversion11/1  "fault"
  Extract Bits/1 -> Data Type Conversion8/1  "limit  switch"
  Extract Bits9/1 -> Data Type Conversion30/1  "limit  switch"
  EtherCAT PDO Receive3/1 -> Extract Bits/1  "Digital inputs []"
  Extract Bits17/1 -> Data Type Conversion27/1
  Extract Bits49/1 -> Data Type Conversion62/1  "fault"
  Extract Bits7/1 -> Data Type Conversion2/1  "STO selected"
  Extract Bits40/1 -> Data Type Conversion52/1  "fault"
  Extract Bits50/1 -> Data Type Conversion61/1  "quick stop"
  Bus Creator25/1 -> Bus Creator22/4  "Fault"
  EtherCAT PDO Receive22/1 -> Data Type Conversion29/1
  Data Type Conversion61/1 -> ?  "quick stop"
  Extract Bits28/1 -> Data Type Conversion45/1  "ready to switch on"
  Extract Bits13/1 -> Data Type Conversion22/1  "fault"
  Data Type Conversion10/1 -> ?  "quick stop"
  Data Type Conversion67/1 -> ?  "HW enabled"
  Data Type Conversion41/1 -> ?
  Data Type Conversion3/1 -> ?  "HW enabled"
  Data Type Conversion57/1 -> ?  "HW enabled"
  Data Type Conversion37/1 -> ?  "HW enabled"
  Data Type Conversion47/1 -> ?  "HW enabled"
  Bus Creator22/1 -> Status/1
  Data Type Conversion21/1 -> ?  "quick stop"

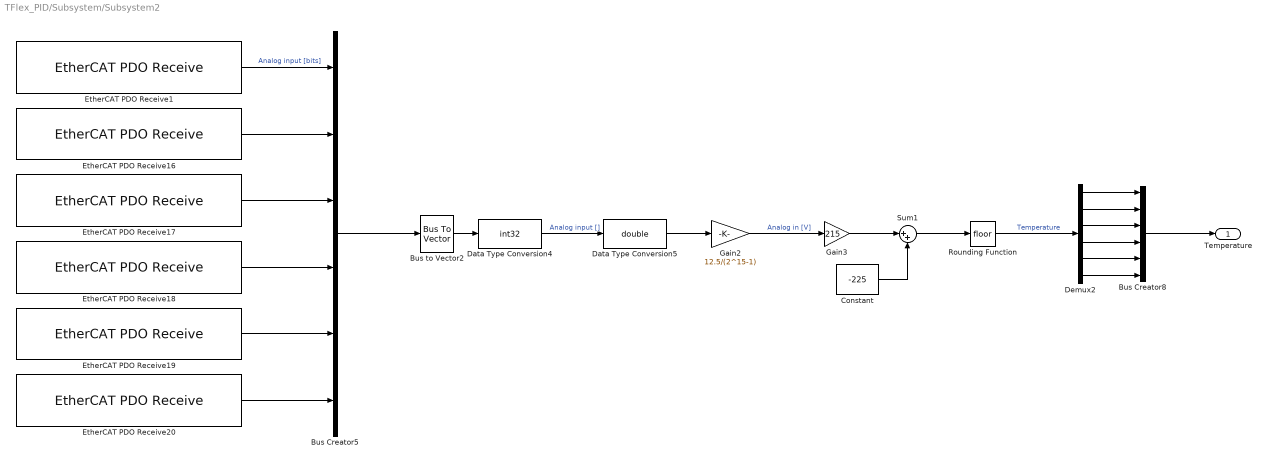
== system TFlex_PID/Subsystem/Subsystem2 ==
  Bus Creator5 : BusCreator  Inputs=6
  Bus Creator8 : BusCreator  Inputs=6
  Bus to Vector2 : BusToVector
  Constant : Constant  Value=-225
  Data Type Conversion4 : DataTypeConversion  OutDataTypeStr=int32
  Data Type Conversion5 : DataTypeConversion  OutDataTypeStr=double
  Demux2 : Demux  Outputs=6
  EtherCAT PDO Receive1 : xpcethercatlib/EtherCAT PDO Receive  Priority=2  sig_name=Drive 2 (AKD).Inputs.AOUT_INPUT_VALUE  sig_offset=480  sig_type=int16  type_size=16  sig_dim=1  device_id=0  sample_time=0.001000
      settings: SourceProductName=Simulink Real-Time  SourceProductBaseCode=XP
  EtherCAT PDO Receive16 : xpcethercatlib/EtherCAT PDO Receive  Priority=2  sig_name=Drive 3 (AKD).Inputs.AOUT_INPUT_VALUE  sig_offset=12512  sig_type=int16  type_size=16  sig_dim=1  device_id=0  sample_time=0.001000
      settings: SourceProductName=Simulink Real-Time  SourceProductBaseCode=XP
  EtherCAT PDO Receive17 : xpcethercatlib/EtherCAT PDO Receive  Priority=2  sig_name=Drive 4 (AKD).Inputs.AOUT_INPUT_VALUE  sig_offset=24800  sig_type=int16  type_size=16  sig_dim=1  device_id=0  sample_time=0.001000
      settings: SourceProductName=Simulink Real-Time  SourceProductBaseCode=XP
  EtherCAT PDO Receive18 : xpcethercatlib/EtherCAT PDO Receive  Priority=2  sig_name=Drive 5 (AKD).Inputs.AOUT_INPUT_VALUE  sig_offset=37088  sig_type=int16  type_size=16  sig_dim=1  device_id=0  sample_time=0.001000
      settings: SourceProductName=Simulink Real-Time  SourceProductBaseCode=XP
  EtherCAT PDO Receive19 : xpcethercatlib/EtherCAT PDO Receive  Priority=2  sig_name=Drive 6 (AKD).Inputs.AOUT_INPUT_VALUE  sig_offset=37248  sig_type=int16  type_size=16  sig_dim=1  device_id=0  sample_time=0.001000
      settings: SourceProductName=Simulink Real-Time  SourceProductBaseCode=XP
  EtherCAT PDO Receive20 : xpcethercatlib/EtherCAT PDO Receive  Priority=2  sig_name=Drive 7 (AKD).Inputs.AOUT_INPUT_VALUE  sig_offset=37408  sig_type=int16  type_size=16  sig_dim=1  device_id=0  sample_time=0.001000
      settings: SourceProductName=Simulink Real-Time  SourceProductBaseCode=XP
  Gain2 : Gain  Gain=12.5/(2^15-1)
  Gain3 : Gain  Gain=215
  Rounding Function : Rounding
  Sum1 : Sum  Inputs=|++  OutDataTypeStr=double
  Temperature : Outport
  wires:
  Rounding Function/1 -> Demux2/1  "Temperature"
  Demux2/1 -> Bus Creator8/1
  Demux2/5 -> Bus Creator8/5
  EtherCAT PDO Receive1/1 -> Bus Creator5/1  "Analog input [bits]"
  Demux2/3 -> Bus Creator8/3
  Data Type Conversion5/1 -> Gain2/1
  EtherCAT PDO Receive17/1 -> Bus Creator5/3
  Bus to Vector2/1 -> Data Type Conversion4/1
  Constant/1 -> Sum1/2
  EtherCAT PDO Receive18/1 -> Bus Creator5/4
  Demux2/2 -> Bus Creator8/2
  EtherCAT PDO Receive19/1 -> Bus Creator5/5
  Demux2/4 -> Bus Creator8/4
  Bus Creator5/1 -> Bus to Vector2/1
  Data Type Conversion4/1 -> Data Type Conversion5/1  "Analog input []"
  EtherCAT PDO Receive16/1 -> Bus Creator5/2
  Sum1/1 -> Rounding Function/1
  Demux2/6 -> Bus Creator8/6
  Bus Creator8/1 -> Temperature/1
  Gain3/1 -> Sum1/1
  Gain2/1 -> Gain3/1  "Analog in [V]"
  EtherCAT PDO Receive20/1 -> Bus Creator5/6

== system TFlex_PID/Update Posterior/Features ==
  x : Inport
  SIGMA : Inport  Port=2
  sf : Inport  Port=3
  D : Inport  Port=4
  Divide2 : Product  Inputs=*/
  Product : Product  Multiplication=Matrix(*)
  Product2 : Product
  Sqrt : Sqrt  SaturateOnIntegerOverflow=on
  Transpose2 : Math  Operator=transpose  SaturateOnIntegerOverflow=on
  Transpose3 : Math  Operator=transpose  SaturateOnIntegerOverflow=on
  Transpose4 : Math  Operator=transpose  SaturateOnIntegerOverflow=on
  Trigonometric Function : Trigonometry  Operator=cos
  Trigonometric Function1 : Trigonometry
  Vector Concatenate1 : Concatenate
  phi_out : Outport
  wires:
  SIGMA/1 -> Product/1
  Product2/1 -> phi_out/1
  D/1 -> Sqrt/1
  Trigonometric Function1/1 -> Transpose3/1
  Trigonometric Function/1 -> Transpose2/1
  sf/1 -> Divide2/1
  Vector Concatenate1/1 -> Transpose4/1
  Transpose3/1 -> Vector Concatenate1/2
  Product/1 -> Trigonometric Function1/1, Trigonometric Function/1
  Divide2/1 -> Product2/1
  Transpose4/1 -> Product2/2
  Sqrt/1 -> Divide2/2
  Transpose2/1 -> Vector Concatenate1/1
  x/1 -> Product/2

== matlab function TFlex_PID/Update Posterior/MATLAB Function ==
  settings: updateMethod=DISCRETE  sampleTime=ts
  data: R input; w_out output; b input; w_init input
function w_out = updateW(R,b,w_init)
persistent w
if(isempty(w))
    w = w_init;
end
%coder.extrinsic('solve_chol');
%w = solve_chol(R,b);
w = R\(R'\b);
w_out = w;

== matlab function TFlex_PID/Update Posterior/MATLAB Function1 ==
  settings: updateMethod=DISCRETE  sampleTime=ts
  data: R_out output; phi input; R_init input
function R_out = cholupdate_fcn(phi,R_init)
persistent R; 
if(isempty(R))
    R = R_init;
end
R = cholupdate(R,phi);
R_out = R;

== matlab function TFlex_PID/Update Posterior/MATLAB Function4 ==
  settings: updateMethod=DISCRETE  sampleTime=ts
  data: update input; b_out output; b_init input
function b_out = updateB(update, b_init)
persistent b 
if(isempty(b))
    b = b_init;
end

b = b + update;
b_out = b;
